simulink model "f_22_stabilator_control"  (R2025b)
settings: Solver=ode15s  StartTime=0.0  StopTime=8  RelTol=1e-3
InitFcn:
  | Running_in_Simulink = 1;
  | 
  | Relation;
  | 
  | EHA_initialization;
values from neighbouring files (symbols this model uses):
  deflection = deflection_min:0.01:deflection_max    [Relation.m]
  extension = sqrt(a^2 + r^2 - 2.*a.*r.*cos(deg2rad(alpha-deflection))) - d    [Relation.m]
  F_act = M_pivot ./ lever_arm_actuator    [Relation.m]
  J = 0.205    [EHA_initialization.m]
  V_actot = 3e-3    (= 0.003)    [EHA_initialization.m]
  V_gasi = V_gasnom    (= 0.00206)    [EHA_initialization.m]
  V_gasnom = 2.06e-3    (= 0.00206)    [EHA_initialization.m]
  velocity = 300    [Relation.m]
undefined symbols (not defined in the file or in its folder): M_eq_array, max_allowed_deflection, min_allowed_deflection
libraries: fl_lib x17, nesl_utility x12, SimscapeFluids_lib x7, simulink x2, ee_lib x1, slpidlib x1
settings Model: Creator=Arseni  LastModifiedBy=Arseni

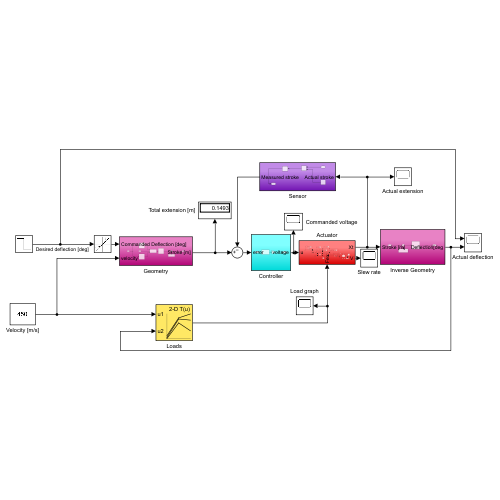
[thumbnail: Simulink's stored preview of the top-level diagram]
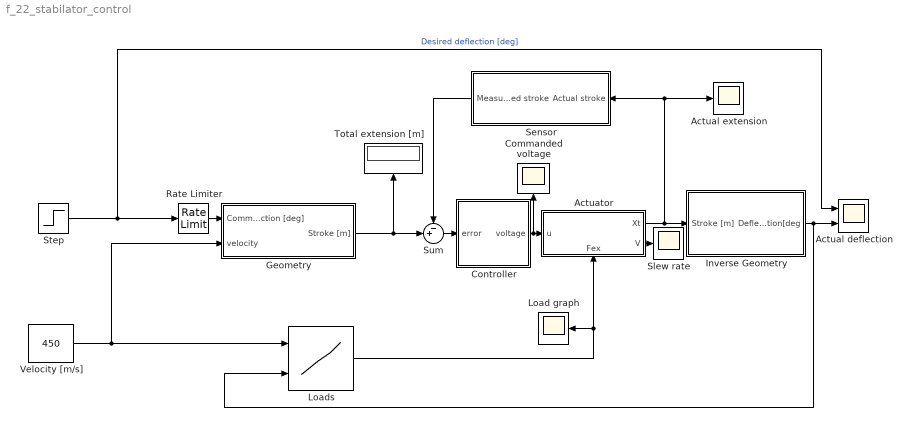
== system f_22_stabilator_control ==
  Actual deflection : Scope  NumInputPorts=2
      settings: ActiveDisplayYMinimum=-23.051092231500004  ActiveDisplayYMaximum=2.7474433984251712  DataLoggingVariableName=ScopeData2
  Actual extension : Scope
      settings: ActiveDisplayYMinimum=-0.46554881704214957  ActiveDisplayYMaximum=0.393661332723093
  Actuator : Subsystem
      settings: PortSchema="{\"entries\":[{\"content\":{\"sides\":[{\"content\":{\"connectorIds\":[\"In1\"]},\"type\":\"ConnectorPlacement.EquallySpacedRectSide\",\"uuid\":\"943d01fe-42c0-45b1-9341-7d812506ef46\"},{\"content\":{\"connectorIds\":[\"Out1\",\"Out2\"],\"side\":\"RIGHT\"},\"type\":\"ConnectorPlacement.EquallySpacedRectSide\",\"uuid\":\"406f4aac-e724-45d2-a2bf-fb82cce20e93\"},{\"content\":{\"side\":\"TOP\"},\"type\":\"ConnectorPlacement.EquallySpacedRectSide\",\"uuid\":\"b2672d80-a78b-4b49-883e-7d4d522a2a85\"},{\"content\":{\"connectorIds\":[\"In2\"],\"side\":\"BOTTOM\"},\"type\":\"ConnectorPlacement.EquallySpacedRectSide\",\"uuid\":\"ce0b7e96-337f-4b82-8a54-268fa65edfc7\"}]},\"type\":\"ConnectorPlacement.EquallySpacedConnector\",\"uuid\":\"852eed82-4be2-4e21-befb-75521b9915fe\"}],\"packageUris\":[\"http://schema.mathworks.com/mf0/Connector/R2020b\"],\"version\":\"1.0\"}"
  Commanded voltage : Scope
      settings: ActiveDisplayYMinimum=-321.13569228196531  ActiveDisplayYMaximum=123.99047438919578  DataLoggingVariableName=ScopeData3
  Controller : Subsystem
  Geometry : Subsystem
  Inverse Geometry : Subsystem
  Load graph : Scope
      settings: ActiveDisplayYMinimum=-639262.39888357045  ActiveDisplayYMaximum=50770.010571138249  DataLoggingVariableName=ScopeData4
  Loads : Lookup_n-D  BreakpointsForDimension1=velocity  BreakpointsForDimension2=deflection  Table=F_act  InternalRulePriority=Speed  RndMeth=Simplest
      settings: InputPortMap=u0,u1
  Rate Limiter : RateLimiter  RisingSlewLimit=60  FallingSlewLimit=-60
  Sensor : Subsystem
  Slew rate : Scope
      settings: ActiveDisplayYMinimum=-0.19699161303203394  ActiveDisplayYMaximum=0.087603872620795789
  Step : Step  Time=3  After=-20  SampleTime=0
  Sum : Sum  Inputs=-+|
  Total extension [m] : Display
  Velocity [m/s] : Constant  Value=450
  wires:
  Step/1 -> Actual deflection/1, Rate Limiter/1  "Desired deflection [deg]"
  Velocity [m/s]/1 -> Loads/1, Geometry/2(velocity)
  Actuator/1(Xt) -> Inverse Geometry/1(Stroke [m]), Actual extension/1, Sensor/1(Actual stroke)
  Actuator/2(V) -> Slew rate/1
  Geometry/1(Stroke [m]) -> Total extension [m]/1, Sum/2
  Sum/1 -> Controller/1(error)
  Loads/1 -> Actuator/2(Fex), Load graph/1
  Inverse Geometry/1(Deflection[deg) -> Loads/2, Actual deflection/2
  Sensor/1(Measured stroke) -> Sum/1
  Controller/1(voltage) -> Actuator/1(u), Commanded voltage/1
  Rate Limiter/1 -> Geometry/1(Commanded Deflection [deg])

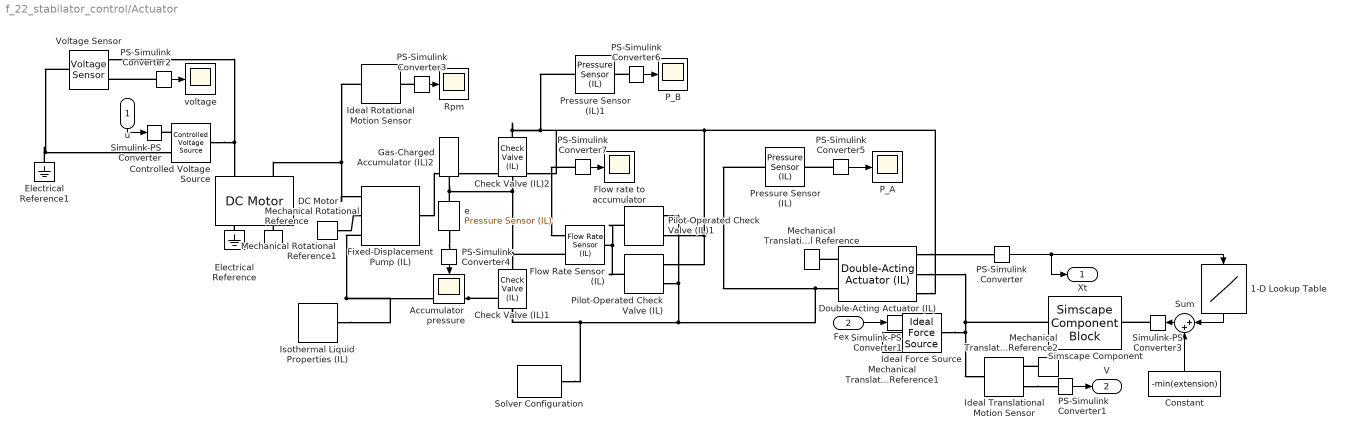
== system f_22_stabilator_control/Actuator ==
  u : Inport
  Fex : Inport  Port=2
  1-D Lookup Table : Lookup_n-D  NumberOfTableDimensions=1  BreakpointsForDimension1=flip(extension)  Table=flip(M_eq_array)  InternalRulePriority=Speed  RndMeth=Simplest
  Accumulator pressure : Scope
      settings: ActiveDisplayYMinimum=2.5372225941755947E+7  ActiveDisplayYMaximum=3.0439462704747144E+7  DataLoggingVariableName=ScopeData7
  Check Valve (IL)1 : SimscapeFluids_lib/Isothermal Liquid/Valves & Orifices/Directional Control Valves/Check Valve (IL)  opening_spec=fluids.isothermal_liquid.valves_orifices.enum.PressureOpeningSpec.Linear  pressure_control_spec=fluids.isothermal_liquid.valves_orifices.enum.pressure_control_spec.dp  p_crack_differential=P_crack MPa  p_crack_gauge=0.1 MPa  press_max_differential=P_omax MPa  press_max_gauge=0.2 MPa  area_max=A_omax m^2  area_leak=A_cleak m^2  p_diff_TLU=[0.01 : 0.01 : 0.1] MPa  valve_area_TLU=[1e-10, 1e-05, 2e-05, 3e-05, 4e-05, 5e-05, 6e-05, 7.5e-05, 8.5e-05, .0001] m^2  vol_flow_TLU=[.000358, .045, .11, .191, .284, .39, .505, .63, .764, .905] .* 1e-3 m^3/s  area=A_cAB m^2  Cd=C_cdis  Re_c=Re_crit  smoothing_factor=F_sm  pressure_recovery=false  opening_dynamics=false  tau=0.1 s
      settings: InternalSimscapePortConfiguration="{\"Bottom\":[],\"Left\":[{\"id\":\"A\",\"label\":\"A\",\"type\":\"foundation.isothermal_liquid.isothermal_liquid\"}],\"Right\":[{\"id\":\"B\",\"label\":\"B\",\"type\":\"foundation.isothermal_liquid.isothermal_liquid\"}],\"Top\":[]}"
  Check Valve (IL)2 : SimscapeFluids_lib/Isothermal Liquid/Valves & Orifices/Directional Control Valves/Check Valve (IL)  opening_spec=fluids.isothermal_liquid.valves_orifices.enum.PressureOpeningSpec.Linear  pressure_control_spec=fluids.isothermal_liquid.valves_orifices.enum.pressure_control_spec.dp  p_crack_differential=P_crack MPa  p_crack_gauge=0.1 MPa  press_max_differential=P_omax MPa  press_max_gauge=0.2 MPa  area_max=A_omax m^2  area_leak=A_cleak m^2  p_diff_TLU=[0.01 : 0.01 : 0.1] MPa  valve_area_TLU=[1e-10, 1e-05, 2e-05, 3e-05, 4e-05, 5e-05, 6e-05, 7.5e-05, 8.5e-05, .0001] m^2  vol_flow_TLU=[.000358, .045, .11, .191, .284, .39, .505, .63, .764, .905] .* 1e-3 m^3/s  area=A_cAB m^2  Cd=C_cdis  Re_c=Re_crit  smoothing_factor=F_sm  pressure_recovery=false  opening_dynamics=false  tau=0.1 s
      settings: InternalSimscapePortConfiguration="{\"Bottom\":[],\"Left\":[{\"id\":\"A\",\"label\":\"A\",\"type\":\"foundation.isothermal_liquid.isothermal_liquid\"}],\"Right\":[{\"id\":\"B\",\"label\":\"B\",\"type\":\"foundation.isothermal_liquid.isothermal_liquid\"}],\"Top\":[]}"
  Constant : Constant  Value=-min(extension)
  Controlled Voltage Source : fl_lib/Electrical/Electrical Sources/Controlled Voltage Source
  DC Motor : ee_lib/Electromechanical/Brushed Motors/DC Motor  field_option=ee.enum.field_option.pm  Rf=100 Ohm  Lf=1 H  Laf=0.15 H  If0=0 A  parameterization=ee.enum.dcparam_option.circuit_param  Ra=R Ohm  La=L H  emf_or_torque=ee.enum.emf_or_torque.kv  Kv=K_e V/rpm  Ki=6.876e-4 N*m/A  T_stall=0.24e-3 N*m  w_max=19100 rpm  w_rated=15000 rpm  P_rated=0.08 W  V_rated=1.5 V  lam_param=ee.enum.lam_param.damping  i_noload=0 A  V_i_noload=1.5 V  J=J kg*m^2  lam=K_vism N*m*s/rad  speed0=W_init rpm  alpha=3.93e-3 1/K  Tmeas=25 degC  thermal_mass=100 J/K  initial_temperature=25 degC
  Double-Acting Actuator (IL) : SimscapeFluids_lib/Isothermal Liquid/Actuators/Double-Acting Actuator (IL)  single_fluid=true  mech_orientation=foundation.enum.MechOrientationTranslational.Positive  piston_area_A=A_cA m^2  piston_area_B=A_cB m^2  stroke=Stroke m  dead_volume_A=V_deadA m^3  dead_volume_B=V_deadB m^3  pressure_spec=foundation.enum.pressure_spec.atmospheric  environment_pressure=0.101325 MPa  hardstop_model=simscape.enum.hardstop.smooth  stiff_coeff=Hard_s N/m  damping_coeff=Hard_d N*s/m  transition=Trans mm  coeff_rest=0.7  v_tol=0.001 m/s  f_tol=0.001 N  cushion_A_spec=false  area_plunger_A=1e-4 m^2  length_plunger_A=1e-3 m  area_cushion_orifice_A=1e-6 m^2  area_leak_plunger_A=1e-7 m^2  p_crack_differential_A=0.01 MPa  press_max_differential_A=0.1 MPa  check_valve_area_max_A=1e-4 m^2  check_valve_area_leak_A=1e-10 m^2  smoothing_factor_A=0.01  cushion_B_spec=false  area_plunger_B=1e-4 m^2  length_plunger_B=1e-3 m  area_cushion_orifice_B=1e-6 m^2  area_leak_plunger_B=1e-7 m^2  p_crack_differential_B=0.01 MPa  press_max_differential_B=0.1 MPa  check_valve_area_max_B=1e-4 m^2  check_valve_area_leak_B=1e-10 m^2  smoothing_factor_B=0.01  friction_spec=true  breakaway_Coulomb_ratio=R_bc  breakaway_velocity=V_brk m/s  preload_force=F_pre N  Coulomb_coeff=C_fc N/Pa  viscous_coeff=C_fv N*s/m  leakage_spec=true  clearance=Clearance m  piston_length=L_head m  displacement_spec=foundation.enum.DisplacementSpec.Calculate  x0=d_ini m  dynamic_compressibility=true  p0_A=P_A MPa  p0_B=P_B MPa  p_nominal_A=0.101325 MPa  p_nominal_B=0.101325 MPa
      settings: InternalSimscapePortConfiguration="{\"Bottom\":[],\"Left\":[{\"id\":\"C\",\"label\":\"C\",\"type\":\"foundation.mechanical.translational.translational\"},{\"id\":\"A\",\"label\":\"A\",\"type\":\"foundation.isothermal_liquid.isothermal_liquid\"}],\"Right\":[{\"id\":\"p_out\",\"label\":\"p\",\"type\":\"output\"},{\"id\":\"R\",\"label\":\"R\",\"type\":\"foundation.mechanical.translational.translational\"},{\"id\":\"B\",\"label\":\"B\",\"type\":\"foundation.isothermal_liquid.isothermal_liquid\"}],\"Top\":[]}"
  Electrical Reference : fl_lib/Electrical/Electrical Elements/Electrical Reference
  Electrical Reference1 : fl_lib/Electrical/Electrical Elements/Electrical Reference
  Fixed-Displacement Pump (IL) : SimscapeFluids_lib/Isothermal Liquid/Pumps & Motors/Fixed-Displacement Pump (IL)  leakage_friction_spec=fluids.isothermal_liquid.pumps_motors.enum.pump_motor_loss_spec.analytical  displacement=D cm^3/rev  omega_nominal=W_nom rpm  p_nominal=P_nom MPa  vol_eff_nominal=eff_V  mech_eff_nominal=eff_M  no_load_torque=T_NL N*m  p_diff_eff_TLU=[.1, 1, 2] MPa  omega_eff_TLU=[250, 500, 1000, 2000, 3000, 4000] rpm  vol_eff_TLU=[.816, .908, .954, .977, .981, .984; .325, .663, .831, .916, .925, .946; .137, .568, .78, .892, .893, .91]  mech_eff_TLU=[.996, .996, .996, .996, .996, .996; .988, .989, .989, .989, .989, .99; .981, .981, .982, .982, .983, .984]  p_diff_loss_TLU=[.1, 1, 2] MPa  omega_loss_TLU=[250, 500, 1000, 2000, 3000, 4000] rpm  vol_loss_TLU=1e-3 * [.023, .023, .023, .023, .0285, .032; .0844, .0842, .0845, .084, .1125, .108; .1079, .108, .11, .108, .1605, .18] m^3/s  mech_loss_TLU=[.002, .002, .002, .002, .002, .002; .0607, .0556, .0556, .0556, .0556, .0505; .1937, .1937, .1833, .1833, .1729, .1626] N*m  vol_eff_min=1e-3  vol_eff_max=1  mech_eff_min=1e-3  mech_eff_max=1  pressure_threshold=1e-3 MPa  omega_threshold=100 rpm  supplied_range_check=simscape.enum.assert.action.none  pump_mode_check=simscape.enum.assert.action.none  pressure_check=simscape.enum.assert.action.none  p_min_valid=0.101325 MPa
      settings: InternalSimscapePortConfiguration="{\"Bottom\":[{\"id\":\"A\",\"label\":\"A\",\"type\":\"foundation.isothermal_liquid.isothermal_liquid\"}],\"Left\":[],\"Right\":[{\"id\":\"R\",\"label\":\"R\",\"type\":\"foundation.mechanical.rotational.rotational\"},{\"id\":\"C\",\"label\":\"C\",\"type\":\"foundation.mechanical.rotational.rotational\"}],\"Top\":[{\"id\":\"B\",\"label\":\"B\",\"type\":\"foundation.isothermal_liquid.isothermal_liquid\"}]}"
  Flow Rate Sensor (IL) : fl_lib/Isothermal Liquid/Sensors/Flow Rate Sensor (IL)  sensor_type=foundation.enum.mass_volumetric_sensor.mass
      settings: InternalSimscapePortConfiguration="{\"Bottom\":[],\"Left\":[{\"id\":\"A\",\"label\":\"A\",\"type\":\"foundation.isothermal_liquid.isothermal_liquid\"}],\"Right\":[{\"id\":\"B\",\"label\":\"B\",\"type\":\"foundation.isothermal_liquid.isothermal_liquid\"},{\"id\":\"M\",\"label\":\"M\",\"type\":\"output\"}],\"Top\":[]}"
  Flow rate to accumulator : Scope
      settings: ActiveDisplayYMinimum=-4.9065043922899125  ActiveDisplayYMaximum=12.518611954613087  DataLoggingVariableName=ScopeData11
  Gas-Charged Accumulator (IL)2 : SimscapeFluids_lib/Isothermal Liquid/Tanks & Accumulators/Gas-Charged Accumulator (IL)  capacity=V_actot m^3  dead_volume=V_gasmin m^3  p_precharge=P_pre MPa  k_sh=hs  stiff_coeff=S_hs MPa/m^3  dynamic_compressibility=true  liquid_volume_specify=on  liquid_volume_priority=High  liquid_volume=V_actot - V_gasi m^3  liquid_volume_nominal_specify=on  liquid_volume_nominal_value=V_actot - V_gasnom  liquid_volume_nominal_unit=m^3  liquid_mass_specify=off  liquid_mass_priority=None  liquid_mass=5 kg  liquid_mass_nominal_specify=off  liquid_mass_nominal_value=1  liquid_mass_nominal_unit=kg  p_I_specify=on  p_I_priority=None  p_I=P_aci MPa  p_I_nominal_specify=on  p_I_nominal_value=P_acnom  p_I_nominal_unit=MPa
      settings: InternalSimscapePortConfiguration="{\"Bottom\":[],\"Left\":[],\"Right\":[{\"id\":\"A\",\"label\":\"A\",\"type\":\"foundation.isothermal_liquid.isothermal_liquid\"}],\"Top\":[]}"
  Ideal Force Source : fl_lib/Mechanical/Mechanical Sources/Ideal Force Source
  Ideal Rotational Motion Sensor : fl_lib/Mechanical/Mechanical Sensors/Ideal Rotational Motion Sensor  reference=foundation.enum.MeasurementReference.absolute  acceleration_port=false  velocity_port=true  position_port=false  wrap_angle=false  offset=0 rad
      settings: InternalSimscapePortConfiguration="{\"Bottom\":[],\"Left\":[{\"id\":\"R\",\"label\":\"R\",\"type\":\"foundation.mechanical.rotational.rotational\"}],\"Right\":[{\"id\":\"W\",\"label\":\"W\",\"type\":\"output\"}],\"Top\":[]}"
  Ideal Translational Motion Sensor : fl_lib/Mechanical/Mechanical Sensors/Ideal Translational Motion Sensor  reference=foundation.enum.MeasurementReference.difference  acceleration_port=false  velocity_port=true  position_port=false  offset=0 m
      settings: InternalSimscapePortConfiguration="{\"Bottom\":[],\"Left\":[{\"id\":\"R\",\"label\":\"R\",\"type\":\"foundation.mechanical.translational.translational\"}],\"Right\":[{\"id\":\"C\",\"label\":\"C\",\"type\":\"foundation.mechanical.translational.translational\"},{\"id\":\"V\",\"label\":\"V\",\"type\":\"output\"}],\"Top\":[]}"
  Isothermal Liquid Properties (IL) : fl_lib/Isothermal Liquid/Utilities/Isothermal Liquid Properties (IL)  rho_L_atm=IL_density kg/m^3  bulk_modulus_model=foundation.enum.bulk_modulus_model.const  beta_gain=6  beta_L_atm=IL_bulk Pa  nu_atm=IL_Kvs m^2/s  p_atm=AP MPa  p_min=P_minv Pa  properties_range_check=simscape.enum.assert.action.error  air_fraction=0.005  polytropic_index=1.0  rho_g_atm=1.225 kg/m^3  air_dissolution_model=false  p_crit=3 MPa
  Mechanical Rotational Reference : fl_lib/Mechanical/Rotational Elements/Mechanical Rotational Reference
  Mechanical Rotational Reference1 : fl_lib/Mechanical/Rotational Elements/Mechanical Rotational Reference
  Mechanical Translational Reference : fl_lib/Mechanical/Translational Elements/Mechanical Translational Reference
  Mechanical Translational Reference1 : fl_lib/Mechanical/Translational Elements/Mechanical Translational Reference
  Mechanical Translational Reference2 : fl_lib/Mechanical/Translational Elements/Mechanical Translational Reference
  PS-Simulink Converter{,1..7} (8 alike) : nesl_utility/PS-Simulink Converter  PhysicalDomain=network_engine_domain  SubClassName=ps_output  LeftPortType=input  RightPortType=output  PseudoPeriodic=off  Frequencies=[]  VectorFormat=inherit  Unit=inherit  AffineConversion=off
  P_A : Scope
      settings: ActiveDisplayYMinimum=1.4163990081753973E+7  ActiveDisplayYMaximum=4.0053533708658643E+7  DataLoggingVariableName=ScopeData9
  P_B : Scope
      settings: ActiveDisplayYMinimum=2.5879183873794913E+7  ActiveDisplayYMaximum=3.4343018444654338E+7  DataLoggingVariableName=ScopeData8
  Pilot-Operated Check Valve (IL) : SimscapeFluids_lib/Isothermal Liquid/Valves & Orifices/Directional Control Valves/Pilot-Operated Check Valve (IL)  pilot_pressure_dir=fluids.isothermal_liquid.valves_orifices.directional_control_valves.enum.PilotPressureDir.open  spool_config=fluids.isothermal_liquid.valves_orifices.directional_control_valves.enum.SpoolConfig.connected  pressure_spec=fluids.isothermal_liquid.valves_orifices.directional_control_valves.enum.pilot_pressure_control_spec.pX_pA  opening_spec=fluids.isothermal_liquid.valves_orifices.enum.PressureOpeningSpec.Linear  p_crack_differential=P_crack MPa  press_max_differential=P_diff_max MPa  p_control_TLU=[0.01 : 0.01 : 0.1] MPa  valve_area_TLU=[1e-10, 1e-05, 2e-05, 3e-05, 4e-05, 5e-05, 6e-05, 7.5e-05, 8.5e-05, .0001] m^2  p_diff_ref_TLU=[0.01 : 0.01 : 0.1] MPa  vol_flow_ref_TLU=[.000358, .045, .11, .191, .284, .39, .505, .63, .764, .905] .* 1e-3 m^3/s  pilot_ratio=Pilot_ratio  area_max=A_max m^2  area_leak=A_pleak m^2  area=inf m^2  Cd=C_pdis  Re_c=Re_pcrit  smoothing_factor=F_psm  pressure_recovery=false  opening_dynamics=false  tau=0.1 s
      settings: InternalSimscapePortConfiguration="{\"Bottom\":[],\"Left\":[{\"id\":\"A\",\"label\":\"A\",\"type\":\"foundation.isothermal_liquid.isothermal_liquid\"},{\"id\":\"X\",\"label\":\"X\",\"type\":\"foundation.isothermal_liquid.isothermal_liquid\"}],\"Right\":[{\"id\":\"B\",\"label\":\"B\",\"type\":\"foundation.isothermal_liquid.isothermal_liquid\"}],\"Top\":[]}"
  Pilot-Operated Check Valve (IL)1 : SimscapeFluids_lib/Isothermal Liquid/Valves & Orifices/Directional Control Valves/Pilot-Operated Check Valve (IL)  pilot_pressure_dir=fluids.isothermal_liquid.valves_orifices.directional_control_valves.enum.PilotPressureDir.open  spool_config=fluids.isothermal_liquid.valves_orifices.directional_control_valves.enum.SpoolConfig.connected  pressure_spec=fluids.isothermal_liquid.valves_orifices.directional_control_valves.enum.pilot_pressure_control_spec.pX_pA  opening_spec=fluids.isothermal_liquid.valves_orifices.enum.PressureOpeningSpec.Linear  p_crack_differential=P_crack MPa  press_max_differential=P_diff_max MPa  p_control_TLU=[0.01 : 0.01 : 0.1] MPa  valve_area_TLU=[1e-10, 1e-05, 2e-05, 3e-05, 4e-05, 5e-05, 6e-05, 7.5e-05, 8.5e-05, .0001] m^2  p_diff_ref_TLU=[0.01 : 0.01 : 0.1] MPa  vol_flow_ref_TLU=[.000358, .045, .11, .191, .284, .39, .505, .63, .764, .905] .* 1e-3 m^3/s  pilot_ratio=1  area_max=A_max m^2  area_leak=A_pleak m^2  area=inf m^2  Cd=C_pdis  Re_c=Re_pcrit  smoothing_factor=F_psm  pressure_recovery=false  opening_dynamics=false  tau=0.1 s
      settings: InternalSimscapePortConfiguration="{\"Bottom\":[],\"Left\":[{\"id\":\"A\",\"label\":\"A\",\"type\":\"foundation.isothermal_liquid.isothermal_liquid\"},{\"id\":\"X\",\"label\":\"X\",\"type\":\"foundation.isothermal_liquid.isothermal_liquid\"}],\"Right\":[{\"id\":\"B\",\"label\":\"B\",\"type\":\"foundation.isothermal_liquid.isothermal_liquid\"}],\"Top\":[]}"
  Pressure Sensor (IL) : fl_lib/Isothermal Liquid/Sensors/Pressure Sensor (IL)  pressure_measure=foundation.enum.pressure_measure.absolute
      settings: InternalSimscapePortConfiguration="{\"Bottom\":[],\"Left\":[{\"id\":\"A\",\"label\":\"A\",\"type\":\"foundation.isothermal_liquid.isothermal_liquid\"}],\"Right\":[{\"id\":\"Pa\",\"label\":\"Pa\",\"type\":\"output\"}],\"Top\":[]}"
  Pressure Sensor (IL)1 : fl_lib/Isothermal Liquid/Sensors/Pressure Sensor (IL)  pressure_measure=foundation.enum.pressure_measure.absolute
      settings: InternalSimscapePortConfiguration="{\"Bottom\":[],\"Left\":[{\"id\":\"A\",\"label\":\"A\",\"type\":\"foundation.isothermal_liquid.isothermal_liquid\"}],\"Right\":[{\"id\":\"Pa\",\"label\":\"Pa\",\"type\":\"output\"}],\"Top\":[]}"
  Rpm : Scope
      settings: ActiveDisplayYMinimum=-135.72537308013966  ActiveDisplayYMaximum=218.6596527314527  DataLoggingVariableName=ScopeData6
  Simscape Component : SimscapeComponentBlock  SourceFile=Variable_mass  ComponentPath=Variable_mass  ComponentVariants="[\"Variable_mass\"]"  ComponentVariantNames="[\"Variable_mass\"]"  ClassName=Variable_mass  SchemaVersion=1  v_specify=off  v_priority=None  v=0 m/s  v_nominal_specify=off  v_nominal_value=1  v_nominal_unit=m/s  f_specify=off  f_priority=None  f=0 N  f_nominal_specify=off  f_nominal_value=1  f_nominal_unit=N
      settings: CopyFcn=simscape.sscblock.internal.componentBlockCallback(gcbh,'COPY')  PreCopyFcn=simscape.sscblock.internal.componentBlockCallback(gcbh,'PRECOPY')  PreDeleteFcn=simscape.sscblock.internal.componentBlockCallback(gcbh,'PREDELETE')  InternalSimscapePortConfiguration="{\"Bottom\":[],\"Left\":[{\"id\":\"R\",\"label\":\"R\",\"type\":\"foundation.mechanical.translational.translational\"}],\"Right\":[{\"id\":\"M_eq\",\"label\":\"M\",\"type\":\"input\"}],\"Top\":[]}"
      mask Type: Variable Mass
  Simulink-PS Converter : nesl_utility/Simulink-PS Converter  PhysicalDomain=network_engine_domain  SubClassName=ps_input  LeftPortType=input  RightPortType=output  PseudoPeriodic=off  Frequencies=[]  NoiseDistribution=none  NoiseParameters=[]  Unit=1  AffineConversion=off  FilteringAndDerivatives=provide  SimscapeFilterOrder=1  InputFilterTimeConstant=0.001  UdotUserProvided=0
  Simulink-PS Converter1 : nesl_utility/Simulink-PS Converter  PhysicalDomain=network_engine_domain  SubClassName=ps_input  LeftPortType=input  RightPortType=output  PseudoPeriodic=off  Frequencies=[]  NoiseDistribution=none  NoiseParameters=[]  Unit=1  AffineConversion=off  FilteringAndDerivatives=provide  SimscapeFilterOrder=1  InputFilterTimeConstant=0.001  UdotUserProvided=0
  Simulink-PS Converter3 : nesl_utility/Simulink-PS Converter  PhysicalDomain=network_engine_domain  SubClassName=ps_input  LeftPortType=input  RightPortType=output  PseudoPeriodic=off  Frequencies=[]  NoiseDistribution=none  NoiseParameters=[]  Unit=1  AffineConversion=off  FilteringAndDerivatives=provide  SimscapeFilterOrder=1  InputFilterTimeConstant=0.001  UdotUserProvided=0
  Solver Configuration : nesl_utility/Solver Configuration  PhysicalDomain=network_engine_domain  SubClassName=solver  LeftPortType=input  RightPortType=generic  Tones=[]  Harmonics=[]  SimulateNoise=off  Profile=off  UseLocalSampling=off  EnableSwitchedLinearOptims=on  FrequencyDomain=off  UseCCode=off  RelTol=0.001  AbsTol=0.001  MinStep=1e-09  ToWorkspace=off  RevertToSquareIcSolve=off  NumHomotopyIterations=100  PhasorMode=off  PhasorModeNumHarmonics=1  ConsistencySolver=NEWTON_XTOL_AFTER_FTOL  IndexReductionMethod=DerivativeReplacement  DoDC=off  ResidualTolerance=1e-09  ConsistencyTolSource=GLOBAL  ConsistencyAbsTol=0.001  ConsistencyRelTol=0.001  ConsistencyTolFactor=0.001  UseLocalSolver=off  LocalSolverChoice=NE_BACKWARD_EULER_ADVANCER  ResolveIndetEquations=on  FunctionEvalNumThread=1  LocalSolverSampleTime=0.001  DoFixedCost=off  MaxNonlinIter=3  MaxModeIter=2  ComputeImpulses=off  ImpulseIterations=2  LinearAlgebra=auto  LinearAlgebraNumThread=0  EquationFormulation=NE_TIME_EF  DelaysMemoryBudget=1024  AutomaticFiltering=on  FilteringTimeConstant=0.001  PartitionStorageMethod=AS_NEEDED  PartitionMemoryBudget=1024  PartitionMethod=ROBUST  MultibodyUseLocalSolver=off  MultibodyLocalSolverChoice=ODE1  MultibodyLocalSolverSampleTime=0.001
  Sum : Sum  Inputs=|++
  Voltage Sensor : fl_lib/Electrical/Electrical Sensors/Voltage Sensor
  e : fl_lib/Isothermal Liquid/Sensors/Pressure Sensor (IL)  pressure_measure=foundation.enum.pressure_measure.absolute
      settings: InternalSimscapePortConfiguration="{\"Bottom\":[],\"Left\":[{\"id\":\"A\",\"label\":\"A\",\"type\":\"foundation.isothermal_liquid.isothermal_liquid\"}],\"Right\":[{\"id\":\"Pa\",\"label\":\"Pa\",\"type\":\"output\"}],\"Top\":[]}"
  voltage : Scope
      settings: ActiveDisplayYMinimum=-203.65637272014231  ActiveDisplayYMaximum=178.12051421815812  DataLoggingVariableName=ScopeData5
  Xt : Outport
  V : Outport  Port=2
  wires:
  u/1 -> Simulink-PS Converter/1
  PS-Simulink Converter/1 -> 1-D Lookup Table/1, Xt/1
  Fex/1 -> Simulink-PS Converter1/1
  PS-Simulink Converter1/1 -> V/1
  1-D Lookup Table/1 -> Sum/1
  Constant/1 -> Sum/2
  Sum/1 -> Simulink-PS Converter3/1
  PS-Simulink Converter2/1 -> voltage/1
  PS-Simulink Converter3/1 -> Rpm/1
  PS-Simulink Converter5/1 -> P_A/1
  PS-Simulink Converter6/1 -> P_B/1
  PS-Simulink Converter4/1 -> Accumulator pressure/1
  PS-Simulink Converter7/1 -> Flow rate to accumulator/1
  connections:
  Fixed-Displacement Pump (IL)/RConn3 -- Isothermal Liquid Properties (IL)/RConn1 -- Check Valve (IL)1/RConn1 -- Pressure Sensor (IL)/LConn1 -- Double-Acting Actuator (IL)/LConn2 -- Pilot-Operated Check Valve (IL)1/LConn2 -- Pilot-Operated Check Valve (IL)/LConn1 -- Solver Configuration/RConn1
  DC Motor/LConn2 -- Ideal Rotational Motion Sensor/LConn1 -- Fixed-Displacement Pump (IL)/RConn1
  Check Valve (IL)2/LConn1 -- Flow Rate Sensor (IL)/RConn1 -- Check Valve (IL)1/LConn1 -- e/LConn1 -- Gas-Charged Accumulator (IL)2/RConn1
  Double-Acting Actuator (IL)/LConn1 -- Mechanical Translational Reference/LConn1
  Pressure Sensor (IL)1/LConn1 -- Pilot-Operated Check Valve (IL)/LConn2 -- Pilot-Operated Check Valve (IL)1/LConn1 -- Double-Acting Actuator (IL)/RConn3 -- Fixed-Displacement Pump (IL)/LConn1 -- Check Valve (IL)2/RConn1
  Mechanical Rotational Reference/LConn1 -- DC Motor/RConn2
  Electrical Reference/LConn1 -- DC Motor/RConn1
  Controlled Voltage Source/RConn1 -- Simulink-PS Converter/RConn1
  Controlled Voltage Source/LConn1 -- Voltage Sensor/RConn2 -- DC Motor/LConn1
  Electrical Reference1/LConn1 -- Controlled Voltage Source/RConn2 -- Voltage Sensor/LConn1
  Double-Acting Actuator (IL)/RConn1 -- PS-Simulink Converter/LConn1
  Mechanical Rotational Reference1/LConn1 -- Fixed-Displacement Pump (IL)/RConn2
  Double-Acting Actuator (IL)/RConn2 -- Simscape Component/LConn1 -- Ideal Translational Motion Sensor/LConn1 -- Ideal Force Source/LConn1
  Ideal Translational Motion Sensor/RConn2 -- PS-Simulink Converter1/LConn1
  Simulink-PS Converter1/RConn1 -- Ideal Force Source/RConn1
  Ideal Force Source/RConn2 -- Mechanical Translational Reference1/LConn1
  Mechanical Translational Reference2/LConn1 -- Ideal Translational Motion Sensor/RConn1
  Simulink-PS Converter3/RConn1 -- Simscape Component/RConn1
  PS-Simulink Converter2/LConn1 -- Voltage Sensor/RConn1
  PS-Simulink Converter3/LConn1 -- Ideal Rotational Motion Sensor/RConn1
  PS-Simulink Converter6/LConn1 -- Pressure Sensor (IL)1/RConn1
  PS-Simulink Converter5/LConn1 -- Pressure Sensor (IL)/RConn1
  e/RConn1 -- PS-Simulink Converter4/LConn1
  Pilot-Operated Check Valve (IL)1/RConn1 -- Pilot-Operated Check Valve (IL)/RConn1 -- Flow Rate Sensor (IL)/LConn1
  PS-Simulink Converter7/LConn1 -- Flow Rate Sensor (IL)/RConn2

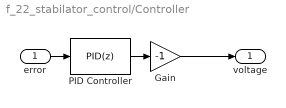
== system f_22_stabilator_control/Controller ==
  error : Inport
  Gain : Gain  Gain=-1
  PID Controller : slpidlib/PID Controller  Controller=PID  Form=Parallel  TimeDomain=Discrete-time  UseExternalTs=off  SampleTime=0.0005  IntegratorMethod=Forward Euler  FilterMethod=Forward Euler  ControllerParametersSource=internal  P=50000  I=50000  UseKiTs=off  D=3000  UseExternalDerivativeSource=off  N=1  UseFilter=on  TunerSelectOption=Transfer Function Based (PID Tuner App)  InitialConditionSource=internal  InitialConditionForIntegrator=0  InitialConditionForFilter=0  DifferentiatorICPrevScaledInput=0  ExternalReset=none  TrackingMode=off  Kt=1  LimitOutput=on  SatLimitsSource=internal  UpperSaturationLimit=292.4  LowerSaturationLimit=-292.4  LinearizeAsGain=off  AntiWindupMode=back-calculation  Kb=1  LimitIntegrator=on  UpperIntegratorSaturationLimit=30  LowerIntegratorSaturationLimit=-30  RndMeth=Nearest  POutMin=[]  POutMax=[]  IOutMin=[]  IOutMax=[]  DOutMin=[]  DOutMax=[]  NOutMin=[]  NOutMax=[]  SumOutMin=[]  SumOutMax=[]  SaturationOutMin=[]  SaturationOutMax=[]  PParamMin=[]  PParamMax=[]  IParamMin=[]  IParamMax=[]  DParamMin=[]  DParamMax=[]  NParamMin=[]  NParamMax=[]  KbParamMin=[]  KbParamMax=[]  KtParamMin=[]  KtParamMax=[]  KbOutMin=[]  KbOutMax=[]  KtOutMin=[]  KtOutMax=[]  IntegratorOutMin=[]  IntegratorOutMax=[]  FilterOutMin=[]  FilterOutMax=[]  SumI1OutMin=[]  SumI1OutMax=[]  SumI2OutMin=[]  SumI2OutMax=[]  SumI3OutMin=[]  SumI3OutMax=[]  SumI4OutMin=[]  SumI4OutMax=[]  SumDOutMin=[]  SumDOutMax=[]  DifferentiatorOutMin=[]  DifferentiatorOutMax=[]  FilterDiffOutCoefMin=[]  FilterDiffOutCoefMax=[]  ReciprocalOutMin=[]  ReciprocalOutMax=[]  SumDenOutMin=[]  SumDenOutMax=[]  SumNumOutMin=[]  SumNumOutMax=[]  DivideOutMin=[]  DivideOutMax=[]  UdiffTsProdOutMin=[]  UdiffTsProdOutMax=[]  NTsProdOutMin=[]  NTsProdOutMax=[]  UintegralTsProdOutMin=[]  UintegralTsProdOutMax=[]  UngainTsProdOutMin=[]  UngainTsProdOutMax=[]  ClampingZeroOutDataTypeStr=Inherit: Inherit via back propagation  ClampingZeroOutMin=[]  ClampingZeroOutMax=[]  FilterDenConstantOutDataTypeStr=Inherit: Inherit via back propagation  FilterDenConstantOutMin=[]  FilterDenConstantOutMax=[]  PCopyOutDataTypeStr=Inherit: Inherit via back propagation  PCopyOutMin=[]  PCopyOutMax=[]  NCopyOutDataTypeStr=Inherit: Inherit via back propagation  NCopyOutMin=[]  NCopyOutMax=[]  IntegratorContinuousStateAttributes=''  IntegratorStateMustResolveToSignalObject=off  IntegratorRTWStateStorageClass=Auto  FilterContinuousStateAttributes=''  FilterStateMustResolveToSignalObject=off  FilterRTWStateStorageClass=Auto  ParallelPVariant=InternalParameters  IdealPVariant=Disabled  IVariant=InternalParameters  DVariant=InternalParameters  IntegratorVariant=Discrete  SatVariant=Enabled  AWVariant=BackCalculation  PCopyVariant=Disabled  TRVariant=Disabled  FdbkBlocksVariant=Forward  IdealPFdbkVariant=Disabled  SatFdbkVariant=Disabled  DerivativeFilterVariant=ForwardEulerFilter  NVariant=InternalParameters  NCopyVariant=Disabled  FilterICVariant=InternalICsFilter  IntegratorICVariant=InternalICs  ExternalResetVariant=Disabled  TRSumVariant=Passthrough  SumFdbkVariant=Disabled  SumVariant=Sum_PID  TsampFilterVariant=InternalTs  TsampNgainVariant=Passthrough  TsampIntegralVariant=Disabled_SignalSpec  ExternalSaturationOutDataTypeStr=Inherit: Same as second input  DerivativeSourceVariant=ErrorSignal  PreIntVariant=InternalPreInt
  voltage : Outport
  wires:
  PID Controller/1 -> Gain/1
  error/1 -> PID Controller/1
  Gain/1 -> voltage/1

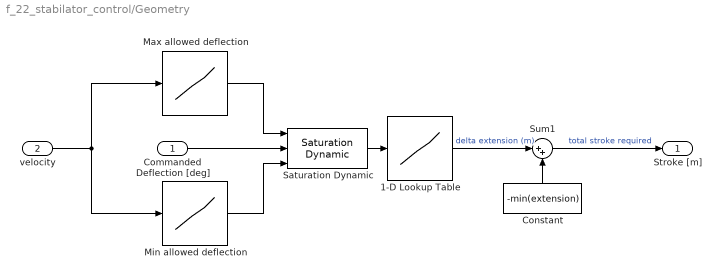
== system f_22_stabilator_control/Geometry ==
  Commanded Deflection [deg] : Inport
  velocity : Inport  Port=2
  1-D Lookup Table : Lookup_n-D  NumberOfTableDimensions=1  BreakpointsForDimension1=deflection  Table=extension  InternalRulePriority=Speed  RndMeth=Simplest
  Constant : Constant  Value=-min(extension)
  Max allowed deflection : Lookup_n-D  NumberOfTableDimensions=1  BreakpointsForDimension1=velocity  Table=max_allowed_deflection  InternalRulePriority=Speed  RndMeth=Simplest
  Min allowed deflection : Lookup_n-D  NumberOfTableDimensions=1  BreakpointsForDimension1=velocity  Table=min_allowed_deflection  InternalRulePriority=Speed  RndMeth=Simplest
  Saturation Dynamic : simulink/Discontinuities/Saturation Dynamic  OutMin=[]  OutMax=[]  OutDataTypeStr=Inherit: Same as second input  OutDataType=fixdt(1, 16)  OutScaling=2^-10  DoSatur=off
  Sum1 : Sum  Inputs=|++
  Stroke [m] : Outport
  wires:
  Constant/1 -> Sum1/2
  1-D Lookup Table/1 -> Sum1/1  "delta extension (m)"
  Sum1/1 -> Stroke [m]/1  "total stroke required"
  Max allowed deflection/1 -> Saturation Dynamic/1
  Min allowed deflection/1 -> Saturation Dynamic/3
  velocity/1 -> Max allowed deflection/1, Min allowed deflection/1
  Commanded Deflection [deg]/1 -> Saturation Dynamic/2
  Saturation Dynamic/1 -> 1-D Lookup Table/1

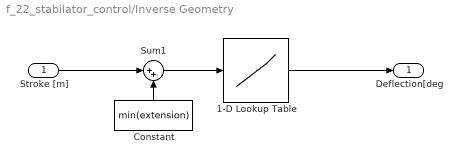
== system f_22_stabilator_control/Inverse Geometry ==
  Stroke [m] : Inport
  1-D Lookup Table : Lookup_n-D  NumberOfTableDimensions=1  BreakpointsForDimension1=flip(extension)  Table=flip(deflection)  InternalRulePriority=Speed  RndMeth=Simplest
  Constant : Constant  Value=min(extension)
  Sum1 : Sum  Inputs=|++
  Deflection[deg : Outport
  wires:
  Constant/1 -> Sum1/2
  Sum1/1 -> 1-D Lookup Table/1
  Stroke [m]/1 -> Sum1/1
  1-D Lookup Table/1 -> Deflection[deg/1

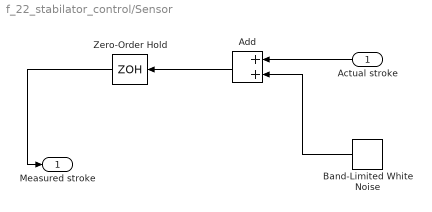
== system f_22_stabilator_control/Sensor ==
  Actual stroke : Inport
  Add : Sum
  Band-Limited White Noise : simulink/Sources/Band-Limited White Noise  Cov=[1e-9]  Ts=0.01  seed=[23341]
  Zero-Order Hold : ZeroOrderHold  SampleTime=0.0005
  Measured stroke : Outport
  wires:
  Zero-Order Hold/1 -> Measured stroke/1
  Actual stroke/1 -> Add/1
  Add/1 -> Zero-Order Hold/1
  Band-Limited White Noise/1 -> Add/2
